simulink model "lftModel"  (R2024a)
settings: Solver=ode1  StartTime=0.0  StopTime=Inf  FixedStep=0.001  RelTol=1e-3
PostLoadFcn:
  | , if any(exist('dsrtsu_mdlpostloadfcn', 'file') ~= 0), dsrtsu_mdlpostloadfcn('Execute', bdroot); end,
InitFcn:
  | , if any(exist('rtifpga_mdlclblib', 'file') ~= 0), rtifpga_mdlclblib('Init', bdroot); end,
undefined symbols (not defined in the file): ampN, Current_Limit, cycles, fb, ff, fHz, fIN, freqs, lc, lcam, Mag_xData, Mag_yData, trajData, wn, xData, yData, z_stroke, z_TDC
libraries: rti1202lib_adc_class1 x7, rti1202lib_dio_class1 x3, simulink x3, rti1202lib_dac_class1 x1
(part 2 of 4)

== system lftModel/Trigger ==
  Trigger Qualisys and Paddles : Inport
  DIO Trigger Paddles : rti1202lib_dio_class1/DIO_CLASS1_BIT_OUT_BL1  DSProperties=struct('RTI',struct('Version',uint32(1),'BlockType',struct('isSLSource',uint8(0),'isSLSink',uint8(1),'isHWSource',uint8(0),'isHWSink',uint8(1),'isSetup',uint8(0),'isInline',uint8(1),'isNonInline',uint8(0),'isInterrupt',uint8(0),'isChannelwise',uint8(1)),'IOBoardType',{{'DS120X','STD','DIOC1'}},'UnitType','BIT','Identifier','BITOUT','DialogType','ML','BlockSet','NONE','SlaveProcessor','NONE'))  RTIBlockInterface=struct('InputPortsWidth',int32(1),'InputPortsActive',1,'InputPortsDataType',{{'SS_BOOLEAN'}},'InputPortsName',{{'In'}},'BlockDisplay',{{['DIO CL1 BIT OUT\nPort: 1\nChannel: 1\nNumber of channels: 1'],'center\'}},'IconTransparency','on','InitLevel',3,'DialogFcn','rti120xstddioc1bitoutgui','BlockName',struct('Token',{{'DIO_CLASS1_BIT_OUT_BL1'}}))  RTIBlockParameters=struct('PortNo',{{1,'OFF',[]}},'ChannelNo',{{1,'OFF',[]}},'ChannelNumOf',{{1,'OFF',[]}},'HighLevel',{{3,'OFF',[1 3]}},'OutputStateInit',{{zeros(1,16),'OFF',[0 1]}},'OutputStateTerm',{{zeros(1,16),'OFF',[0 1]}},'TerminationMode',{{0,'OFF',[0 1]}},'OutputStateTermValidate',{{0,'OFF',[0 1]}},'OutputStateInitSetAll',{{0,'OFF',[0 1]}},'OutputStateTermSetAll',{{0,'OFF',[0 1]}},'EnableEvent',{{0,'OFF',[0 1]}},'EventMode',{{1,'OFF',[1 3]}},'EventOnFalling',{{1,'OFF',[0 1]}},'EventOnRising',{{0,'OFF',[0 1]}},'EventDelay',{{'0','OFF',[0 1.34]}},'EventRate',{{'1','OFF',[1 256]}},'EventBuildCheck',{{false,'OFF',[]}},'TriggerLine',{{1,'OFF',[1 16]}},'EventChannelNoIdx',{{1,'OFF',[1 16]}},'TLCFileName',{{'rti120xdio_c1_bit_out','OFF',[]}})  RTISFcnParameters=struct('PortNo','int16','ChannelNo','int16','ChannelNumOf','int16','HighLevel','int16','OutputStateInit','int16','OutputStateTerm','int16','TerminationMode','int16','OutputStateTermValidate','int16','EnableEvent','int16','EventMode','int16','EventOnFalling','int16','EventOnRising','int16','EventDelay','double','EventRate','int16','TriggerLine','int16','EventChannelNoIdx','int16','TLCFileName','char')  RTIBlockParaDefault=struct('PortNo',1,'ChannelNo',1,'ChannelNumOf',1,'HighLevel',1,'OutputStateInit',zeros(1,16),'OutputStateTerm',zeros(1,16),'TerminationMode',0,'OutputStateTermValidate',0,'OutputStateInitSetAll',0,'OutputStateTermSetAll',0,'EnableEvent',0,'EventMode',1,'EventOnFalling',1,'EventOnRising',0,'EventDelay',0,'EventRate',1,'EventBuildCheck',0,'TriggerLine',1,'EventChannelNoIdx',1,'TLCFileName','rti120xdio_c1_bit_out')
  DIO Trigger Qualisys : rti1202lib_dio_class1/DIO_CLASS1_BIT_OUT_BL1  DSProperties=struct('RTI',struct('Version',uint32(1),'BlockType',struct('isSLSource',uint8(0),'isSLSink',uint8(1),'isHWSource',uint8(0),'isHWSink',uint8(1),'isSetup',uint8(0),'isInline',uint8(1),'isNonInline',uint8(0),'isInterrupt',uint8(0),'isChannelwise',uint8(1)),'IOBoardType',{{'DS120X','STD','DIOC1'}},'UnitType','BIT','Identifier','BITOUT','DialogType','ML','BlockSet','NONE','SlaveProcessor','NONE'))  RTIBlockInterface=struct('InputPortsWidth',int32(1),'InputPortsActive',1,'InputPortsDataType',{{'SS_BOOLEAN'}},'InputPortsName',{{'In'}},'BlockDisplay',{{['DIO CL1 BIT OUT\nPort: 1\nChannel: 2\nNumber of channels: 1'],'center\'}},'IconTransparency','on','InitLevel',3,'DialogFcn','rti120xstddioc1bitoutgui','BlockName',struct('Token',{{'DIO_CLASS1_BIT_OUT_BL1'}}))  RTIBlockParameters=struct('PortNo',{{1,'OFF',[]}},'ChannelNo',{{2,'OFF',[]}},'ChannelNumOf',{{1,'OFF',[]}},'HighLevel',{{3,'OFF',[1 3]}},'OutputStateInit',{{zeros(1,16),'OFF',[0 1]}},'OutputStateTerm',{{zeros(1,16),'OFF',[0 1]}},'TerminationMode',{{0,'OFF',[0 1]}},'OutputStateTermValidate',{{0,'OFF',[0 1]}},'OutputStateInitSetAll',{{0,'OFF',[0 1]}},'OutputStateTermSetAll',{{0,'OFF',[0 1]}},'EnableEvent',{{0,'OFF',[0 1]}},'EventMode',{{1,'OFF',[1 3]}},'EventOnFalling',{{1,'OFF',[0 1]}},'EventOnRising',{{0,'OFF',[0 1]}},'EventDelay',{{'0','OFF',[0 1.34]}},'EventRate',{{'1','OFF',[1 256]}},'EventBuildCheck',{{false,'OFF',[]}},'TriggerLine',{{1,'OFF',[1 16]}},'EventChannelNoIdx',{{1,'OFF',[1 16]}},'TLCFileName',{{'rti120xdio_c1_bit_out','OFF',[]}})  RTISFcnParameters=struct('PortNo','int16','ChannelNo','int16','ChannelNumOf','int16','HighLevel','int16','OutputStateInit','int16','OutputStateTerm','int16','TerminationMode','int16','OutputStateTermValidate','int16','EnableEvent','int16','EventMode','int16','EventOnFalling','int16','EventOnRising','int16','EventDelay','double','EventRate','int16','TriggerLine','int16','EventChannelNoIdx','int16','TLCFileName','char')  RTIBlockParaDefault=struct('PortNo',1,'ChannelNo',1,'ChannelNumOf',1,'HighLevel',1,'OutputStateInit',zeros(1,16),'OutputStateTerm',zeros(1,16),'TerminationMode',0,'OutputStateTermValidate',0,'OutputStateInitSetAll',0,'OutputStateTermSetAll',0,'EnableEvent',0,'EventMode',1,'EventOnFalling',1,'EventOnRising',0,'EventDelay',0,'EventRate',1,'EventBuildCheck',0,'TriggerLine',1,'EventChannelNoIdx',1,'TLCFileName','rti120xdio_c1_bit_out')
  Trigger Qualisys : DataTypeConversion  OutDataTypeStr=boolean  SaturateOnIntegerOverflow=off  RndMeth=Floor
  Trigger Wavemaker : DataTypeConversion  OutDataTypeStr=boolean  SaturateOnIntegerOverflow=off  RndMeth=Floor
  Use Qualisys : Gain  Gain=0
  Use Wavemaker : Gain  Gain=0
  wires:
  Trigger Wavemaker/1 -> DIO Trigger Paddles/1
  Trigger Qualisys/1 -> DIO Trigger Qualisys/1
  Use Qualisys/1 -> Trigger Qualisys/1
  Use Wavemaker/1 -> Trigger Wavemaker/1
  Trigger Qualisys and Paddles/1 -> Use Qualisys/1, Use Wavemaker/1

== system lftModel/VC Voltage Sense ==
  Gain : Gain  Gain=10.2
  VC Voltage : rti1202lib_adc_class1/ADC_CLASS1_BL1  DSProperties=struct('RTI',struct('Version',uint32(1),'BlockType',struct('isSLSource',uint8(1),'isSLSink',uint8(1),'isHWSource',uint8(0),'isHWSink',uint8(1),'isSetup',uint8(0),'isInline',uint8(1),'isNonInline',uint8(0),'isInterrupt',uint8(0),'isChannelwise',uint8(1)),'IOBoardType',{{'DS120X','STD','ADCC1'}},'UnitType','ADC','Identifier','ADC','DialogType','ML','BlockSet','NONE','SlaveProcessor','NONE'))  RTIBlockInterface=struct('InputPortsActive',0,'InputPortsWidth',int32(1),'InputPortsDataType',{{'SS_BOOLEAN'}},'InputPortsName',{{'Continue'}},'OutputPortsActive',[1 0],'OutputPortsWidth',int32([1 1]),'OutputPortsDataType',{{'SS_DOUBLE','SS_INT16'}},'OutputPortsName',{{'ADC','Status'}},'DialogFcn','rti120xstdadcc1adcgui','SampleTime',{{-1}},'InitLevel',3,'IconTransparency','on','BlockDisplay',{{['ADC CL1\nChannel: 4'],'center'}},'BlockName',struct('Token',{{'ADC_CLASS1_BL1'}}))  RTIBlockParameters=struct('ReadMode',{{1,'OFF',[1 2]}},'ChannelNo',{{4,'OFF',[]}},'ConversionMode',{{1,'OFF',[1 2]}},'TriggerSource',{{1,'OFF',[1 2]}},'TriggerLineIn',{{1,'OFF',[1 16]}},'SampleMode',{{1,'OFF',[1 2]}},'BurstTriggerSource',{{1,'OFF',[1 2]}},'BurstTriggerLine',{{1,'OFF',[1 16]}},'ConvTriggerSource',{{3,'OFF',[1 3]}},'ConvTriggerLine',{{1,'OFF',[1 16]}},'ConvPeriod',{{'100e-6','OFF',[1e-6 1.34]}},'ConvPeriodCheck',{{0,'OFF',[]}},'BurstSize',{{'10','OFF',[]}},'BurstSizeCheck',{{0,'OFF',[]}},'DataSetOffset',{{'0','OFF',[]}},'DataSetOffsetCheck',{{0,'OFF',[]}},'DataSetLength',{{'1','OFF',[]}},'DataSetLengthCheck',{{0,'OFF',[]}},'EnableTriggerEvent',{{0,'OFF',[0 1]}},'TriggerMode',{{2,'OFF',[1 3]}},'TriggerLineOut',{{1,'OFF',[1 16]}},'ADCSWStartEnable',{{0,'OFF',[0 1]}},'SampleTime',{{'-1','OFF',[-1 inf]}},'SampleTimeCheck',{{1,'OFF',[]}},'StatusPortEnable',{{0,'OFF',[0 1]}},'TLCFileName',{{'rti120xadc_c1_adc','OFF',[]}})  RTISFcnParameters=struct('ReadMode','int16','ChannelNo','int16','ConversionMode','int16','TriggerSource','int16','TriggerLineIn','int16','SampleMode','int16','BurstTriggerSource','int16','BurstTriggerLine','int16','ConvTriggerSource','int16','ConvTriggerLine','int16','ConvPeriod','double','BurstSize','int16','DataSetOffset','int16','DataSetLength','int16','EnableTriggerEvent','int16','TriggerMode','int16','TriggerLineOut','int16','ADCSWStartEnable','int16','SampleTime','double','StatusPortEnable','int16','TLCFileName','char')  RTIBlockParaDefault=struct('ReadMode',1,'ChannelNo',1,'ConversionMode',1,'TriggerSource',1,'TriggerLineIn',1,'SampleMode',1,'BurstTriggerSource',1,'BurstTriggerLine',1,'ConvTriggerSource',3,'ConvTriggerLine',1,'ConvPeriod',0.0001,'ConvPeriodCheck',0,'BurstSize',10,'BurstSizeCheck',0,'DataSetOffset',0,'DataSetOffsetCheck',0,'DataSetLength',1,'DataSetLengthCheck',0,'EnableTriggerEvent',0,'TriggerMode',2,'TriggerLineOut',1,'ADCSWStartEnable',0,'SampleTime',-1,'SampleTimeCheck',1,'StatusPortEnable',0,'TLCFileName','rti120xadc_c1_adc')
  dSPACE Gain : Gain  Gain=10
  "Measured VC, Volt " : Outport
  wires:
  VC Voltage/1 -> dSPACE Gain/1
  dSPACE Gain/1 -> Gain/1
  Gain/1 -> "Measured VC, Volt "/1

== system lftModel/Accelerometer/Triggered Subsystem ==
  In1 : Inport
  Trigger : TriggerPort  VariantControl=(inherit)
  Data Store Write : DataStoreWrite  DataStoreName=Vo  IndexOptions=Index vector (dialog)  Indices=1  OutputSizes=1
  wires:
  In1/1 -> Data Store Write/1

== system lftModel/Draft Force /Lookup - Slope ==
  "Position Input, mm" : Inport
  Lookup with Linear Lagrange Interpolation : Lookup_n-D  NumberOfTableDimensions=1  BreakpointsForDimension1=xData  Table=yData  InterpMethod=Linear Lagrange  InternalRulePriority=Speed  RndMeth=Simplest
  Slope (N/amp) : Outport
  wires:
  Lookup with Linear Lagrange Interpolation/1 -> Slope (N/amp)/1
  "Position Input, mm"/1 -> Lookup with Linear Lagrange Interpolation/1

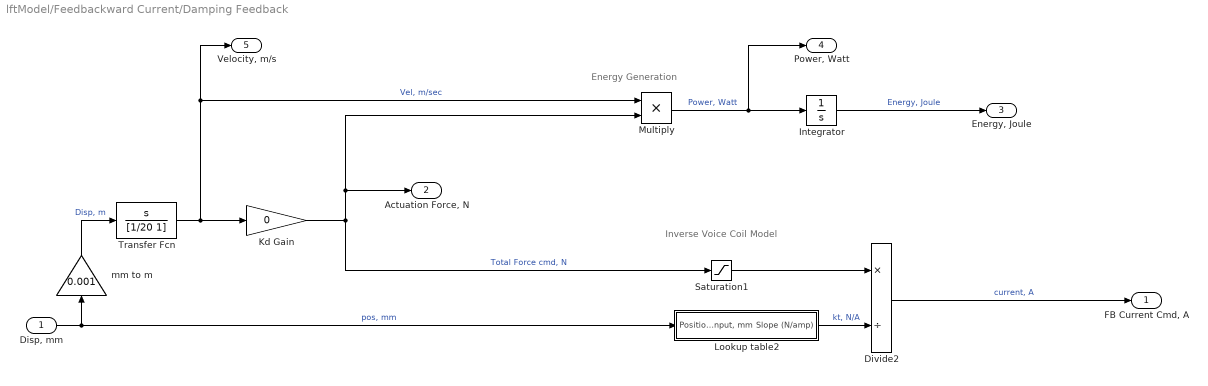
== system lftModel/Feedbackward Current/Damping Feedback ==
  note: Energy Generation
  note: Inverse Voice Coil Model
  "Disp, mm" : Inport
  Divide2 : Product  Inputs=*/
  Integrator : Integrator
  Kd Gain : Gain  Gain=0
  Lookup table2 : Subsystem
  Multiply : Product  Inputs=**
  Saturation1 : Saturate  UpperLimit=fIN.Forcemax  LowerLimit=-fIN.Forcemax
  Transfer Fcn : TransferFcn  Numerator=[1 0]  Denominator=[1/20 1]
  mm to m : Gain  Gain=0.001
  "FB Current Cmd, A" : Outport
  "Actuation Force, N" : Outport  Port=2
  "Energy, Joule " : Outport  Port=3
  "Power, Watt" : Outport  Port=4
  "Velocity, m/s" : Outport  Port=5
  wires:
  Saturation1/1 -> Divide2/1
  Kd Gain/1 -> Saturation1/1, Multiply/2, "Actuation Force, N"/1  "Total Force cmd, N"
  Lookup table2/1(Slope (N/amp)) -> Divide2/2  "kt, N/A"
  Divide2/1 -> "FB Current Cmd, A"/1  "current, A"
  "Disp, mm"/1 -> Lookup table2/1("Position Input, mm"), mm to m/1  "pos, mm"
  Transfer Fcn/1 -> "Velocity, m/s"/1, Multiply/1, Kd Gain/1  "Vel, m/sec"
  mm to m/1 -> Transfer Fcn/1  "Disp, m"
  Multiply/1 -> "Power, Watt"/1, Integrator/1  "Power, Watt"
  Integrator/1 -> "Energy, Joule "/1  "Energy, Joule"

== system lftModel/Feedbackward Current/Velocity Feedback ==
  "Disp, mm" : Inport
  Kv : Gain  Gain=fb.k
  LCAM Gain : Gain  Gain=lcam.gain
  d/dt : Derivative
  "FB Current Cmd, A" : Outport
  wires:
  "Disp, mm"/1 -> Kv/1
  Kv/1 -> d/dt/1
  d/dt/1 -> LCAM Gain/1
  LCAM Gain/1 -> "FB Current Cmd, A"/1

== system lftModel/Feedbackward Current/Zero ==
  "Disp, mm" : Inport
  Gain : Gain  Gain=0
  "FB Current Cmd, A" : Outport
  wires:
  "Disp, mm"/1 -> Gain/1
  Gain/1 -> "FB Current Cmd, A"/1

== system lftModel/Feedforward/Constant ==
  Button Press : Inport
  Time : Inport  Port=2
  "Current Cmd, A" : Gain  Gain=0
  Terminator : Terminator
  smoother : TransferFcn  Numerator=2  Denominator=[1 2]
  smoother1 : TransferFcn  Numerator=2  Denominator=[1 2]
  "Smoothed Current Cmd, A" : Outport
  wires:
  "Current Cmd, A"/1 -> smoother/1
  smoother/1 -> smoother1/1
  smoother1/1 -> "Smoothed Current Cmd, A"/1
  Button Press/1 -> "Current Cmd, A"/1
  Time/1 -> Terminator/1

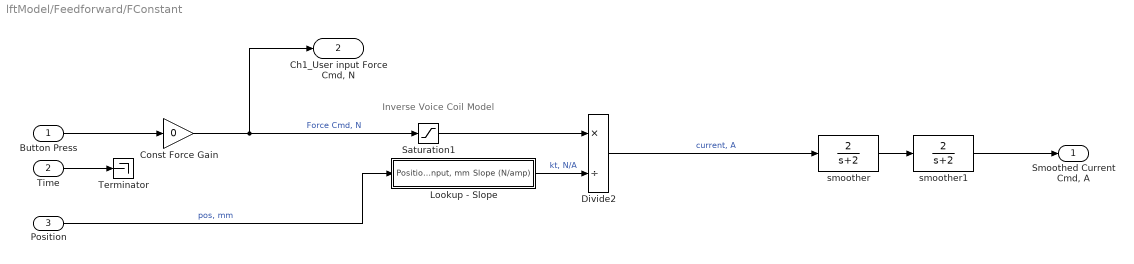
== system lftModel/Feedforward/FConstant ==
  note: Inverse Voice Coil Model
  Button Press : Inport
  Time : Inport  Port=2
  Position : Inport  Port=3
  Const Force Gain : Gain  Gain=0
  Divide2 : Product  Inputs=*/
  Lookup - Slope : Subsystem
  Saturation1 : Saturate  UpperLimit=fIN.Forcemax  LowerLimit=-fIN.Forcemax
  Terminator : Terminator
  smoother : TransferFcn  Numerator=2  Denominator=[1 2]
  smoother1 : TransferFcn  Numerator=2  Denominator=[1 2]
  "Smoothed Current Cmd, A" : Outport
  "Ch1_User input Force Cmd, N" : Outport  Port=2
  wires:
  smoother/1 -> smoother1/1
  Button Press/1 -> Const Force Gain/1
  Time/1 -> Terminator/1
  Divide2/1 -> smoother/1  "current, A"
  Saturation1/1 -> Divide2/1
  Const Force Gain/1 -> "Ch1_User input Force Cmd, N"/1, Saturation1/1  "Force Cmd, N"
  Position/1 -> Lookup - Slope/1("Position Input, mm")  "pos, mm"
  Lookup - Slope/1(Slope (N/amp)) -> Divide2/2  "kt, N/A"
  smoother1/1 -> "Smoothed Current Cmd, A"/1

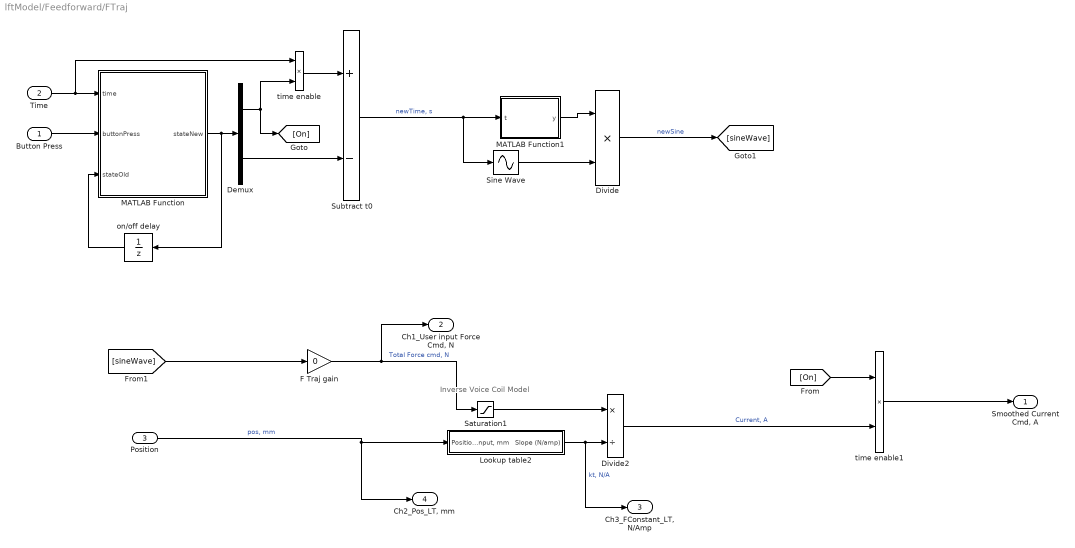
== system lftModel/Feedforward/FTraj  ==
  note: Inverse Voice Coil Model
  Button Press : Inport
  Time : Inport  Port=2
  Position : Inport  Port=3
  Demux : Demux  Outputs=2
  Divide : Product  Inputs=**
  Divide2 : Product  Inputs=*/
  F Traj gain : Gain  Gain=0
  Lookup table2 : Subsystem
  MATLAB Function : MATLAB Function  TreatAsAtomicUnit=on
  MATLAB Function1 : MATLAB Function  TreatAsAtomicUnit=on
  Saturation1 : Saturate  UpperLimit=fIN.Forcemax  LowerLimit=-fIN.Forcemax
  Sine Wave : Sin  TimeSource=Use external signal  Amplitude=ampN  Frequency=fHz*2*pi  SampleTime=0
  Subtract t0 : Sum  Inputs=+-
  on/off delay : UnitDelay  InitialCondition=[0, 0]  SampleTime=-1  HasFrameUpgradeWarning=on
      settings: AttributesFormatString=IC: %<X0>
  time enable : Product  Inputs=**
  time enable1 : Product  Inputs=**
  "Smoothed Current Cmd, A" : Outport
  "Ch1_User input Force Cmd, N" : Outport  Port=2
  "Ch3_FConstant_LT, N/Amp" : Outport  Port=3
  "Ch2_Pos_LT, mm" : Outport  Port=4
  wires:
  on/off delay/1 -> MATLAB Function/3(stateOld)
  Button Press/1 -> MATLAB Function/2(buttonPress)
  Time/1 -> time enable/1, MATLAB Function/1(time)
  MATLAB Function/1(stateNew) -> on/off delay/1, Demux/1
  time enable/1 -> Subtract t0/1
  Demux/1 -> [On], time enable/2
  Demux/2 -> Subtract t0/2
  [On] -> time enable1/1
  Position/1 -> Lookup table2/1("Position Input, mm"), "Ch2_Pos_LT, mm"/1  "pos, mm"
  [sineWave] -> F Traj gain/1
  Lookup table2/1(Slope (N/amp)) -> "Ch3_FConstant_LT, N/Amp"/1, Divide2/2  "kt, N/A"
  Divide2/1 -> time enable1/2  "Current, A"
  Saturation1/1 -> Divide2/1
  time enable1/1 -> "Smoothed Current Cmd, A"/1
  F Traj gain/1 -> "Ch1_User input Force Cmd, N"/1, Saturation1/1  "Total Force cmd, N"
  MATLAB Function1/1(y) -> Divide/1
  Sine Wave/1 -> Divide/2
  Divide/1 -> [sineWave]  "newSine"
  Subtract t0/1 -> Sine Wave/1, MATLAB Function1/1(t)  "newTime, s"
